simulink model "sm_forklift"  (R2021b)
settings: Solver=ode15s  StartTime=0.0  StopTime=53  MaxStep=1e-2  RelTol=1e-3  AbsTol=1e-3  EnableMultiTasking=on
model workspace: external: MATLAB File sm_forklift_parameters.m (data not in the file)
values from neighbouring files (symbols this model uses):
  g = 9.8    [sm_forklift_parameters.m]
undefined symbols (not defined in the file or in its folder): backRest, box, bump, chassis, fork, infPlane, main_mast, pulley, smiData, tire, top_mast, wheel, X, Y, Z
libraries: sm_lib x1413, nesl_utility x83, fl_lib x23, sm_backhoe_lib x6, SignalEditorBlockLib x1
(part 3 of 24)

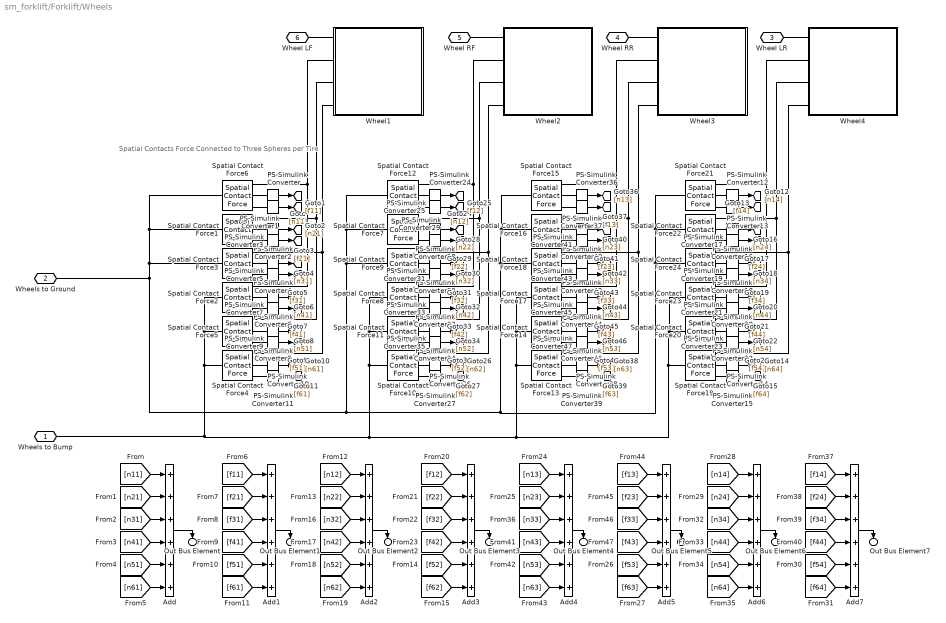
== system sm_forklift/Forklift/Wheels ==
  note: Spatial Contacts Force
      | Connected to Three Spheres per Tire
  Add{,1..7} (8 alike) : Sum  Inputs=++++++
  PS-Simulink Converter{,1..47} (48 alike) : nesl_utility/PS-Simulink Converter  PhysicalDomain=network_engine_domain  SubClassName=ps_output  LeftPortType=input  RightPortType=output  PseudoPeriodic=off  Frequencies=[]  Unit=inherit  AffineConversion=off
      settings: SourceProductBaseCode=PW,SS
  Spatial Contact Force{1..24} (24 alike) : sm_lib/Forces and Torques/Spatial Contact Force  CoefficientOfDynamicFriction=wDynamic  CoefficientOfStaticFriction=wStatic  SenseContactBaseRotation=off  SenseContactBaseTranslation=off  NormalDamping=wDamping  NormalDampingUnits=N/(m/s)  SenseContactFollowerRotation=off  SenseContactFollowerTranslation=off  SenseContactSignal=off  NormalStiffness=wStiffness  NormalStiffnessUnits=N/m  FrictionalCriticalVelocity=wCritical  FrictionalCriticalVelocityUnits=m/s  ZeroCrossDetectContactStartAndEnd=off  FrictionType=SmoothStickSlip  SenseFrictionalForceMagnitude=on  SenseNormalForceMagnitude=on  NormalForceType=SmoothSpringDamper  SenseNormalVelocity=off  SenseSeparationDistance=off  SenseTangentialVelocity=off  SenseTangentialVelocityMagnitude=off  NormalTransitionRegionWidth=wTransWidth  NormalTransitionRegionWidthUnits=mm
  Wheel1 : Subsystem  mask(Wheel){Rwheel=wRadius, Rtire=TireRadius, Raxle=wAxle, W=wWidth, Nc=wResolution, tireColor=TireColor, rhoTire=TireDensity, wheelColor=wColor, rhoWheel=wDensity}
      mask prompts: Rwheel "Wheel Radius (m)"; Rtire "Tire Radius (m)"; Raxle "Axle Radius (m)"; W "Wheel Width (m)"; Nc "Circle Resolution (pts/rev)"; tireColor "Tire Color"; rhoTire "Tire Density (kg/m^3)"; wheelColor "Wheel Color"; rhoWheel "Wheel Density (kg/m^3)"
      mask help:
      | Consists of the backhoe wheel assembly.
      |
      | Attachment points are:
      | A: The center of the wheel's axle.
      mask init:
      | % Circles
      | angles = (0:Nc)' * 2 * pi / Nc;
      | unit_circle = [cos(angles) sin(angles)];
      | unit_circle_cw = flipud(unit_circle);
      | 
      | % Wheel
      | wheelPoints = [Rwheel * unit_circle; Raxle * unit_circle_cw];
      | 
      | % Tire
      | tirePoints = [Rtire * unit_circle; Rwheel * unit_circle_cw];
      | 
      | % Rim
      | H = W*0.15;
      | k = H/(Rwheel^2);
      | vec = linspace(Rwheel,Raxle,10)';
      | rimPoints = [Raxle 0; vec  H-k*vec.^2];
      mask DialogControl ParameterTabVar0 Prompt: General
      mask DialogControl ParameterTabVar01 Prompt: Material Properties
      mask Display:
      | image(repmat(imread(fullfile(matlabroot,'toolbox','physmod','sm','smdemos','backhoe','images','sm_backhoe_wheel.png')),[1 1 3]));
      | port_label('lconn',1,'A');
  Wheel2 : Subsystem  mask(Wheel){Rwheel=wRadius, Rtire=TireRadius, Raxle=wAxle, W=wWidth, Nc=wResolution, tireColor=TireColor, rhoTire=TireDensity, wheelColor=wColor, rhoWheel=wDensity}
      mask prompts: Rwheel "Wheel Radius (m)"; Rtire "Tire Radius (m)"; Raxle "Axle Radius (m)"; W "Wheel Width (m)"; Nc "Circle Resolution (pts/rev)"; tireColor "Tire Color"; rhoTire "Tire Density (kg/m^3)"; wheelColor "Wheel Color"; rhoWheel "Wheel Density (kg/m^3)"
      mask help:
      | Consists of the backhoe wheel assembly.
      |
      | Attachment points are:
      | A: The center of the wheel's axle.
      mask init: same as sm_forklift/Forklift/Wheels/Wheel1
      mask DialogControl ParameterTabVar0 Prompt: General
      mask DialogControl ParameterTabVar01 Prompt: Material Properties
      mask Display:
      | image(repmat(imread(fullfile(matlabroot,'toolbox','physmod','sm','smdemos','backhoe','images','sm_backhoe_wheel.png')),[1 1 3]));
      | port_label('lconn',1,'A');
  Wheel3 : Subsystem  mask(Wheel){Rwheel=wRadius, Rtire=TireRadius, Raxle=wAxle, W=wWidth, Nc=wResolution, tireColor=TireColor, rhoTire=TireDensity, wheelColor=wColor, rhoWheel=wDensity}
      mask prompts: Rwheel "Wheel Radius (m)"; Rtire "Tire Radius (m)"; Raxle "Axle Radius (m)"; W "Wheel Width (m)"; Nc "Circle Resolution (pts/rev)"; tireColor "Tire Color"; rhoTire "Tire Density (kg/m^3)"; wheelColor "Wheel Color"; rhoWheel "Wheel Density (kg/m^3)"
      mask help:
      | Consists of the backhoe wheel assembly.
      |
      | Attachment points are:
      | A: The center of the wheel's axle.
      mask init: same as sm_forklift/Forklift/Wheels/Wheel1
      mask DialogControl ParameterTabVar0 Prompt: General
      mask DialogControl ParameterTabVar01 Prompt: Material Properties
      mask Display:
      | image(repmat(imread(fullfile(matlabroot,'toolbox','physmod','sm','smdemos','backhoe','images','sm_backhoe_wheel.png')),[1 1 3]));
      | port_label('lconn',1,'A');
  Wheel4 : Subsystem  mask(Wheel){Rwheel=wRadius, Rtire=TireRadius, Raxle=wAxle, W=wWidth, Nc=wResolution, tireColor=TireColor, rhoTire=TireDensity, wheelColor=wColor, rhoWheel=wDensity}
      mask prompts: Rwheel "Wheel Radius (m)"; Rtire "Tire Radius (m)"; Raxle "Axle Radius (m)"; W "Wheel Width (m)"; Nc "Circle Resolution (pts/rev)"; tireColor "Tire Color"; rhoTire "Tire Density (kg/m^3)"; wheelColor "Wheel Color"; rhoWheel "Wheel Density (kg/m^3)"
      mask help:
      | Consists of the backhoe wheel assembly.
      |
      | Attachment points are:
      | A: The center of the wheel's axle.
      mask init: same as sm_forklift/Forklift/Wheels/Wheel1
      mask DialogControl ParameterTabVar0 Prompt: General
      mask DialogControl ParameterTabVar01 Prompt: Material Properties
      mask Display:
      | image(repmat(imread(fullfile(matlabroot,'toolbox','physmod','sm','smdemos','backhoe','images','sm_backhoe_wheel.png')),[1 1 3]));
      | port_label('lconn',1,'A');
  Wheels to Bump : PMIOPort  Side=Right
  Wheels to Ground : PMIOPort  Port=2  Side=Right
  Wheel LR : PMIOPort  Port=3  Side=Left
  Wheel RR : PMIOPort  Port=4  Side=Left
  Wheel RF : PMIOPort  Port=5  Side=Left
  Wheel LF : PMIOPort  Port=6  Side=Left
  Out Bus Element : Outport  PortName=S  Element=NomalForce_WheelLF
  Out Bus Element1 : Outport  PortName=S  Element=FrictionalForce_WheelLF
  Out Bus Element2 : Outport  PortName=S  Element=NomalForce_WheelRF
  Out Bus Element3 : Outport  PortName=S  Element=FrictionalForce_WheelRF
  Out Bus Element4 : Outport  PortName=S  Element=NomalForce_WheelRR
  Out Bus Element5 : Outport  PortName=S  Element=FrictionalForce_WheelRR
  Out Bus Element6 : Outport  PortName=S  Element=NomalForce_WheelLR
  Out Bus Element7 : Outport  PortName=S  Element=FrictionalForce_WheelLR
  wires:
  PS-Simulink Converter/1 -> [n11]
  PS-Simulink Converter1/1 -> [f11]
  PS-Simulink Converter3/1 -> [f21]
  PS-Simulink Converter2/1 -> [n21]
  PS-Simulink Converter4/1 -> [n31]
  PS-Simulink Converter5/1 -> [f31]
  PS-Simulink Converter7/1 -> [f41]
  PS-Simulink Converter6/1 -> [n41]
  PS-Simulink Converter8/1 -> [n51]
  PS-Simulink Converter9/1 -> [f51]
  PS-Simulink Converter11/1 -> [f61]
  PS-Simulink Converter10/1 -> [n61]
  PS-Simulink Converter14/1 -> [n64]
  PS-Simulink Converter15/1 -> [f64]
  PS-Simulink Converter23/1 -> [f54]
  PS-Simulink Converter22/1 -> [n54]
  PS-Simulink Converter20/1 -> [n44]
  PS-Simulink Converter21/1 -> [f44]
  PS-Simulink Converter19/1 -> [f34]
  PS-Simulink Converter18/1 -> [n34]
  PS-Simulink Converter16/1 -> [n24]
  PS-Simulink Converter17/1 -> [f24]
  PS-Simulink Converter13/1 -> [f14]
  PS-Simulink Converter12/1 -> [n14]
  PS-Simulink Converter24/1 -> [n12]
  PS-Simulink Converter25/1 -> [f12]
  PS-Simulink Converter29/1 -> [f22]
  PS-Simulink Converter28/1 -> [n22]
  PS-Simulink Converter30/1 -> [n32]
  PS-Simulink Converter31/1 -> [f32]
  PS-Simulink Converter33/1 -> [f42]
  PS-Simulink Converter32/1 -> [n42]
  PS-Simulink Converter34/1 -> [n52]
  PS-Simulink Converter35/1 -> [f52]
  PS-Simulink Converter27/1 -> [f62]
  PS-Simulink Converter26/1 -> [n62]
  PS-Simulink Converter36/1 -> [n13]
  PS-Simulink Converter37/1 -> [f13]
  PS-Simulink Converter41/1 -> [f23]
  PS-Simulink Converter40/1 -> [n23]
  PS-Simulink Converter42/1 -> [n33]
  PS-Simulink Converter43/1 -> [f33]
  PS-Simulink Converter45/1 -> [f43]
  PS-Simulink Converter44/1 -> [n43]
  PS-Simulink Converter46/1 -> [n53]
  PS-Simulink Converter47/1 -> [f53]
  PS-Simulink Converter39/1 -> [f63]
  PS-Simulink Converter38/1 -> [n63]
  [n11] -> Add/1
  [n21] -> Add/2
  [n31] -> Add/3
  [n41] -> Add/4
  [n51] -> Add/5
  [n61] -> Add/6
  [f11] -> Add1/1
  [f31] -> Add1/3
  [f51] -> Add1/5
  [f21] -> Add1/2
  [f41] -> Add1/4
  [f61] -> Add1/6
  [n12] -> Add2/1
  [n22] -> Add2/2
  [n32] -> Add2/3
  [n42] -> Add2/4
  [n52] -> Add2/5
  [n62] -> Add2/6
  [f12] -> Add3/1
  [f22] -> Add3/2
  [f32] -> Add3/3
  [f42] -> Add3/4
  [f52] -> Add3/5
  [f62] -> Add3/6
  [f64] -> Add7/6
  [f54] -> Add7/5
  [f44] -> Add7/4
  [f34] -> Add7/3
  [f24] -> Add7/2
  [f14] -> Add7/1
  [n64] -> Add6/6
  [n54] -> Add6/5
  [n44] -> Add6/4
  [n34] -> Add6/3
  [n24] -> Add6/2
  [n14] -> Add6/1
  [f63] -> Add5/6
  [f43] -> Add5/4
  [f23] -> Add5/2
  [f53] -> Add5/5
  [f33] -> Add5/3
  [f13] -> Add5/1
  [n63] -> Add4/6
  [n53] -> Add4/5
  [n43] -> Add4/4
  [n33] -> Add4/3
  [n23] -> Add4/2
  [n13] -> Add4/1
  Add/1 -> Out Bus Element/1
  Add1/1 -> Out Bus Element1/1
  Add2/1 -> Out Bus Element2/1
  Add3/1 -> Out Bus Element3/1
  Add4/1 -> Out Bus Element4/1
  Add5/1 -> Out Bus Element5/1
  Add6/1 -> Out Bus Element6/1
  Add7/1 -> Out Bus Element7/1
  connections:
  Spatial Contact Force20/LConn1 -- Spatial Contact Force23/LConn1 -- Spatial Contact Force19/LConn1 -- Spatial Contact Force13/LConn1 -- Spatial Contact Force14/LConn1 -- Spatial Contact Force17/LConn1 -- Spatial Contact Force10/LConn1 -- Spatial Contact Force11/LConn1 -- Spatial Contact Force8/LConn1 -- Spatial Contact Force4/LConn1 -- Spatial Contact Force5/LConn1 -- Spatial Contact Force2/LConn1 -- Wheels to Bump/RConn1
  Spatial Contact Force22/LConn1 -- Spatial Contact Force21/LConn1 -- Spatial Contact Force24/LConn1 -- Spatial Contact Force18/LConn1 -- Spatial Contact Force16/LConn1 -- Spatial Contact Force15/LConn1 -- Spatial Contact Force9/LConn1 -- Spatial Contact Force12/LConn1 -- Spatial Contact Force7/LConn1 -- Spatial Contact Force3/LConn1 -- Spatial Contact Force1/LConn1 -- Spatial Contact Force6/LConn1 -- Wheels to Ground/RConn1
  Wheel4/LConn3 -- Spatial Contact Force22/RConn1 -- Spatial Contact Force20/RConn1
  Wheel1/LConn3 -- Spatial Contact Force5/RConn1 -- Spatial Contact Force1/RConn1
  Wheel3/LConn2 -- Spatial Contact Force17/RConn1 -- Spatial Contact Force15/RConn1
  Wheel4/LConn2 -- Spatial Contact Force23/RConn1 -- Spatial Contact Force21/RConn1
  Wheel1/LConn2 -- Spatial Contact Force2/RConn1 -- Spatial Contact Force6/RConn1
  Wheel4/LConn1 -- Wheel LR/RConn1
  Wheel2/LConn3 -- Spatial Contact Force11/RConn1 -- Spatial Contact Force7/RConn1
  Wheel4/LConn4 -- Spatial Contact Force24/RConn1 -- Spatial Contact Force19/RConn1
  Wheel1/LConn4 -- Spatial Contact Force4/RConn1 -- Spatial Contact Force3/RConn1
  Wheel2/LConn4 -- Spatial Contact Force10/RConn1 -- Spatial Contact Force9/RConn1
  Wheel3/LConn4 -- Spatial Contact Force18/RConn1 -- Spatial Contact Force13/RConn1
  Wheel2/LConn2 -- Spatial Contact Force12/RConn1 -- Spatial Contact Force8/RConn1
  Wheel3/LConn3 -- Spatial Contact Force16/RConn1 -- Spatial Contact Force14/RConn1
  Wheel2/LConn1 -- Wheel RF/RConn1
  Wheel1/LConn1 -- Wheel LF/RConn1
  Wheel3/LConn1 -- Wheel RR/RConn1
  Spatial Contact Force12/RConn2 -- PS-Simulink Converter24/LConn1
  Spatial Contact Force7/RConn2 -- PS-Simulink Converter28/LConn1
  Spatial Contact Force7/RConn3 -- PS-Simulink Converter29/LConn1
  Spatial Contact Force9/RConn2 -- PS-Simulink Converter30/LConn1
  Spatial Contact Force9/RConn3 -- PS-Simulink Converter31/LConn1
  Spatial Contact Force8/RConn2 -- PS-Simulink Converter32/LConn1
  Spatial Contact Force8/RConn3 -- PS-Simulink Converter33/LConn1
  Spatial Contact Force11/RConn2 -- PS-Simulink Converter34/LConn1
  Spatial Contact Force11/RConn3 -- PS-Simulink Converter35/LConn1
  PS-Simulink Converter/LConn1 -- Spatial Contact Force6/RConn2
  Spatial Contact Force6/RConn3 -- PS-Simulink Converter1/LConn1
  Spatial Contact Force1/RConn2 -- PS-Simulink Converter2/LConn1
  Spatial Contact Force3/RConn2 -- PS-Simulink Converter4/LConn1
  Spatial Contact Force3/RConn3 -- PS-Simulink Converter5/LConn1
  Spatial Contact Force1/RConn3 -- PS-Simulink Converter3/LConn1
  Spatial Contact Force2/RConn2 -- PS-Simulink Converter6/LConn1
  Spatial Contact Force2/RConn3 -- PS-Simulink Converter7/LConn1
  Spatial Contact Force5/RConn2 -- PS-Simulink Converter8/LConn1
  Spatial Contact Force5/RConn3 -- PS-Simulink Converter9/LConn1
  Spatial Contact Force4/RConn2 -- PS-Simulink Converter10/LConn1
  Spatial Contact Force4/RConn3 -- PS-Simulink Converter11/LConn1
  Spatial Contact Force19/RConn3 -- PS-Simulink Converter15/LConn1
  Spatial Contact Force19/RConn2 -- PS-Simulink Converter14/LConn1
  Spatial Contact Force20/RConn3 -- PS-Simulink Converter23/LConn1
  Spatial Contact Force23/RConn3 -- PS-Simulink Converter21/LConn1
  Spatial Contact Force23/RConn2 -- PS-Simulink Converter20/LConn1
  Spatial Contact Force24/RConn3 -- PS-Simulink Converter19/LConn1
  Spatial Contact Force22/RConn2 -- PS-Simulink Converter16/LConn1
  Spatial Contact Force22/RConn3 -- PS-Simulink Converter17/LConn1
  Spatial Contact Force21/RConn2 -- PS-Simulink Converter12/LConn1
  Spatial Contact Force21/RConn3 -- PS-Simulink Converter13/LConn1
  Spatial Contact Force20/RConn2 -- PS-Simulink Converter22/LConn1
  Spatial Contact Force24/RConn2 -- PS-Simulink Converter18/LConn1
  Spatial Contact Force12/RConn3 -- PS-Simulink Converter25/LConn1
  Spatial Contact Force10/RConn2 -- PS-Simulink Converter26/LConn1
  Spatial Contact Force10/RConn3 -- PS-Simulink Converter27/LConn1
  Spatial Contact Force18/RConn2 -- PS-Simulink Converter42/LConn1
  Spatial Contact Force14/RConn2 -- PS-Simulink Converter46/LConn1
  Spatial Contact Force15/RConn3 -- PS-Simulink Converter37/LConn1
  Spatial Contact Force15/RConn2 -- PS-Simulink Converter36/LConn1
  Spatial Contact Force16/RConn2 -- PS-Simulink Converter40/LConn1
  Spatial Contact Force17/RConn2 -- PS-Simulink Converter44/LConn1
  Spatial Contact Force16/RConn3 -- PS-Simulink Converter41/LConn1
  Spatial Contact Force17/RConn3 -- PS-Simulink Converter45/LConn1
  Spatial Contact Force14/RConn3 -- PS-Simulink Converter47/LConn1
  Spatial Contact Force13/RConn2 -- PS-Simulink Converter38/LConn1
  Spatial Contact Force13/RConn3 -- PS-Simulink Converter39/LConn1
  Spatial Contact Force18/RConn3 -- PS-Simulink Converter43/LConn1

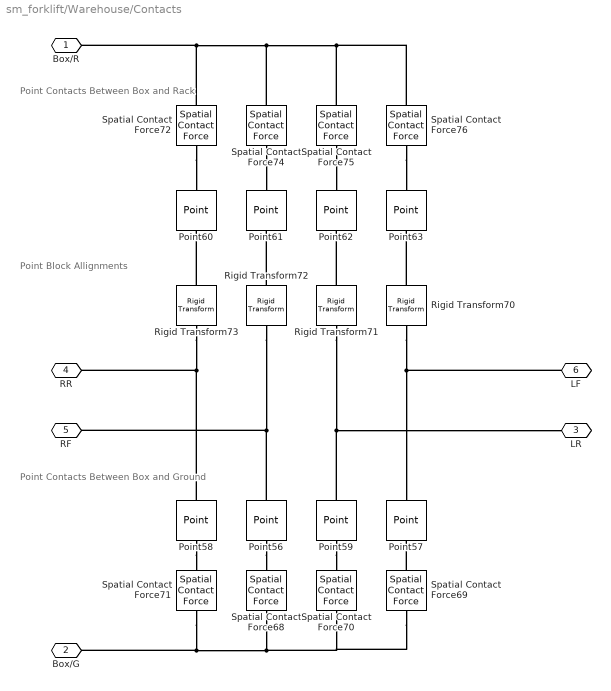
== system sm_forklift/Warehouse/Contacts ==
  note: Point Block Allignments
  note: Point Contacts
      | Between Box and
      | Ground
  note: Point Contacts
      | Between Box and
      | Rack
  Point{56..63} (8 alike) : sm_lib/Curves and Surfaces/Point  GraphicType=None  MarkerShape=Sphere  MarkerSize=10  GraphicVisPropType=SimpleVisualProperties  GraphicDiffuseColor=[0.5 0.5 0.5]  GraphicOpacity=1.0  GraphicSpecularColor=[0.5 0.5 0.5 1.0]  GraphicAmbientColor=[0.15 0.15 0.15 1.0]  GraphicEmissiveColor=[0.0 0.0 0.0 1.0]  GraphicShininess=75
      settings: SourceProductBaseCode=MS
  Rigid Transform70 : sm_lib/Frames and Transforms/Rigid Transform  TranslationMethod=StandardAxis  TranslationStandardOffset=0.2  TranslationLengthUnit=m  TranslationStandardAxis=+X  TranslationCartesianOffset=[0 0 0]  TranslationROffset=0  TranslationROffsetUnits=m  TranslationZOffset=0  TranslationZOffsetUnits=m  TranslationThetaOffset=0  TranslationThetaOffsetUnits=deg  RotationMethod=None  RotationAngleUnits=deg  RotationStandardAxis=+Z  RotationAngle=0.0  RotationArbitraryAxis=[0 0 1]  FollAlignAxisA=+X  BaseAlignAxisA=+Y  FollAlignAxisB=+Y  BaseAlignAxisB=+Z  RotationSequenceAxes=FollowerAxes  RotationSequence=XYX  RotationSequenceAngles=[0 0 0]  RotationSequenceAnglesUnits=deg  RotationMatrix=[1 0 0; 0 1 0; 0 0 1]
  Rigid Transform71 : sm_lib/Frames and Transforms/Rigid Transform  TranslationMethod=StandardAxis  TranslationStandardOffset=0.2  TranslationLengthUnit=m  TranslationStandardAxis=-X  TranslationCartesianOffset=[0 0 0]  TranslationROffset=0  TranslationROffsetUnits=m  TranslationZOffset=0  TranslationZOffsetUnits=m  TranslationThetaOffset=0  TranslationThetaOffsetUnits=deg  RotationMethod=None  RotationAngleUnits=deg  RotationStandardAxis=+Z  RotationAngle=0.0  RotationArbitraryAxis=[0 0 1]  FollAlignAxisA=+X  BaseAlignAxisA=+Y  FollAlignAxisB=+Y  BaseAlignAxisB=+Z  RotationSequenceAxes=FollowerAxes  RotationSequence=XYX  RotationSequenceAngles=[0 0 0]  RotationSequenceAnglesUnits=deg  RotationMatrix=[1 0 0; 0 1 0; 0 0 1]
  Rigid Transform72 : sm_lib/Frames and Transforms/Rigid Transform  TranslationMethod=StandardAxis  TranslationStandardOffset=0.2  TranslationLengthUnit=m  TranslationStandardAxis=+X  TranslationCartesianOffset=[0 0 0]  TranslationROffset=0  TranslationROffsetUnits=m  TranslationZOffset=0  TranslationZOffsetUnits=m  TranslationThetaOffset=0  TranslationThetaOffsetUnits=deg  RotationMethod=None  RotationAngleUnits=deg  RotationStandardAxis=+Z  RotationAngle=0.0  RotationArbitraryAxis=[0 0 1]  FollAlignAxisA=+X  BaseAlignAxisA=+Y  FollAlignAxisB=+Y  BaseAlignAxisB=+Z  RotationSequenceAxes=FollowerAxes  RotationSequence=XYX  RotationSequenceAngles=[0 0 0]  RotationSequenceAnglesUnits=deg  RotationMatrix=[1 0 0; 0 1 0; 0 0 1]
  Rigid Transform73 : sm_lib/Frames and Transforms/Rigid Transform  TranslationMethod=StandardAxis  TranslationStandardOffset=0.2  TranslationLengthUnit=m  TranslationStandardAxis=-X  TranslationCartesianOffset=[0 0 0]  TranslationROffset=0  TranslationROffsetUnits=m  TranslationZOffset=0  TranslationZOffsetUnits=m  TranslationThetaOffset=0  TranslationThetaOffsetUnits=deg  RotationMethod=None  RotationAngleUnits=deg  RotationStandardAxis=+Z  RotationAngle=0.0  RotationArbitraryAxis=[0 0 1]  FollAlignAxisA=+X  BaseAlignAxisA=+Y  FollAlignAxisB=+Y  BaseAlignAxisB=+Z  RotationSequenceAxes=FollowerAxes  RotationSequence=XYX  RotationSequenceAngles=[0 0 0]  RotationSequenceAnglesUnits=deg  RotationMatrix=[1 0 0; 0 1 0; 0 0 1]
  Spatial Contact Force{68..72,74..76} (8 alike) : sm_lib/Forces and Torques/Spatial Contact Force  CoefficientOfDynamicFriction=0.3  CoefficientOfStaticFriction=0.5  SenseContactBaseRotation=off  SenseContactBaseTranslation=off  NormalDamping=1e5  NormalDampingUnits=N/(m/s)  SenseContactFollowerRotation=off  SenseContactFollowerTranslation=off  SenseContactSignal=off  NormalStiffness=1e6  NormalStiffnessUnits=N/m  FrictionalCriticalVelocity=1e-3  FrictionalCriticalVelocityUnits=m/s  ZeroCrossDetectContactStartAndEnd=off  FrictionType=SmoothStickSlip  SenseFrictionalForceMagnitude=off  SenseNormalForceMagnitude=off  NormalForceType=SmoothSpringDamper  SenseNormalVelocity=off  SenseSeparationDistance=off  SenseTangentialVelocity=off  SenseTangentialVelocityMagnitude=off  NormalTransitionRegionWidth=1e-4  NormalTransitionRegionWidthUnits=m
  Box/R : PMIOPort  Side=Left
  Box/G : PMIOPort  Port=2  Side=Left
  LR : PMIOPort  Port=3  Side=Right
  RR : PMIOPort  Port=4  Side=Right
  RF : PMIOPort  Port=5  Side=Right
  LF : PMIOPort  Port=6  Side=Right
  connections:
  Spatial Contact Force71/LConn1 -- Box/G/RConn1 -- Spatial Contact Force69/LConn1 -- Spatial Contact Force70/LConn1 -- Spatial Contact Force68/LConn1
  Point56/LConn1 -- Rigid Transform72/LConn1 -- RF/RConn1
  Point58/RConn1 -- Spatial Contact Force71/RConn1
  Spatial Contact Force72/LConn1 -- Spatial Contact Force76/LConn1 -- Spatial Contact Force75/LConn1 -- Spatial Contact Force74/LConn1 -- Box/R/RConn1
  Point59/LConn1 -- Rigid Transform71/LConn1 -- LR/RConn1
  Spatial Contact Force72/RConn1 -- Point60/RConn1
  Rigid Transform71/RConn1 -- Point62/LConn1
  Point59/RConn1 -- Spatial Contact Force70/RConn1
  Rigid Transform70/RConn1 -- Point63/LConn1
  Rigid Transform73/RConn1 -- Point60/LConn1
  Spatial Contact Force69/RConn1 -- Point57/RConn1
  Point56/RConn1 -- Spatial Contact Force68/RConn1
  Spatial Contact Force75/RConn1 -- Point62/RConn1
  Spatial Contact Force76/RConn1 -- Point63/RConn1
  Rigid Transform70/LConn1 -- LF/RConn1 -- Point57/LConn1
  Point58/LConn1 -- Rigid Transform73/LConn1 -- RR/RConn1
  Rigid Transform72/RConn1 -- Point61/LConn1
  Spatial Contact Force74/RConn1 -- Point61/RConn1

== system sm_forklift/Warehouse/Lift Box ==
  Box : sm_lib/Body Elements/Brick Solid  GraphicAmbientColor=[0.15 0.15 0.15 1.0]  BasedOnType=Mass  BrickDimensions=boxDimensions  BrickDimensionUnits=m  CenterOfMass=[0 0 0]  CenterOfMassUnits=m  GraphicDiffuseColor=boxColor  Density=100  DensityUnits=kg/m^3  DoExposeReferenceFrame=off  GraphicEmissiveColor=[0.0 0.0 0.0 1.0]  ExportEntireGeometry=off  SerializedFrames=<Frames><Frame><Id>Frame1</Id><Value><Name>F1</Name><Origin><Source>GeometricFeature</Source><FeatureName>-z surface</FeatureName></Origin><PrimaryAxis><DefinedDirection>-Z</DefinedDirection><Source>GeometricFeature</Source><SourceDirection>+Z</SourceDirection><FeatureName>-z surface</FeatureName></PrimaryAxis><SecondaryAxis><DefinedDirection>+X</DefinedDirection><Source>ReferenceFrame</Source><SourceDirection>+X</SourceDirection><FeatureName></FeatureName></SecondaryAxis></Value></Frame></Frames>  MarkerShape=Sphere  MarkerSize=10  GraphicType=FromGeometry  InertiaType=CalculateFromGeometry  Mass=boxMass  MassUnits=kg  MomentsOfInertia=[1 1 1]  MomentsOfInertiaUnits=kg*m^2  GraphicOpacity=1.0  ProductsOfInertia=[0 0 0]  ProductsOfInertiaUnits=kg*m^2  GraphicShininess=75  GraphicSpecularColor=[0.5 0.5 0.5 1.0]  GraphicVisPropType=SimpleVisualProperties
  Box Base : sm_lib/Body Elements/File Solid  ExtGeomFileName=Palette_800x1200.step  UnitType=FromFile  ExtGeomFileUnits=m  StepReaderType=HEX  ExportConvexHullGeometry=off  InertiaType=CalculateFromGeometry  Mass=1  MassUnits=kg  CenterOfMass=[0 0 0]  CenterOfMassUnits=m  MomentsOfInertia=[1 1 1]  MomentsOfInertiaUnits=kg*m^2  ProductsOfInertia=[0 0 0]  ProductsOfInertiaUnits=kg*m^2  BasedOnType=Density  Density=bpDensity  DensityUnits=kg/m^3  DoExposeReferenceFrame=on  SerializedFrames=<Frames><Frame><Id>Frame1</Id><Value><Name>LR</Name><Origin><Source>GeometricFeature</Source><FeatureName>point 357</FeatureName></Origin><PrimaryAxis><DefinedDirection>+Z</DefinedDirection><Source>ReferenceFrame</Source><SourceDirection>+Z</SourceDirection><FeatureName></FeatureName></PrimaryAxis><SecondaryAxis><DefinedDirection>+X</DefinedDirection><Source>ReferenceFrame</Source><SourceDirection>+X</SourceDirection><FeatureName></FeatureName></SecondaryAxis></Value></Frame><Frame><Id>Frame2</Id><Value><Name>RR</Name><Origin><Source>GeometricFeature</Source><FeatureName>point 165</FeatureName></Origin><PrimaryAxis><DefinedDirection>+Z</DefinedDirection><Source>ReferenceFrame</Source><SourceDirection>+Z</SourceDirection><FeatureName></FeatureName></PrimaryAxis><SecondaryAxis><DefinedDirection>+X</DefinedDirection><Source>ReferenceFrame</Source><SourceDirection>+X</SourceDirection><FeatureName></FeatureName></SecondaryAxis></Value></Frame><Frame><Id>Frame3</Id><Value><Name>LF</Name><Origin><Source>GeometricFeature</Source><FeatureName>point 358</FeatureName></Origin><PrimaryAxis><DefinedDirection>+Z</DefinedDirection><Source>ReferenceFrame</Source><SourceDirection>+Z</SourceDirection><FeatureName></FeatureName></PrimaryAxis><SecondaryAxis><DefinedDirection>+X</DefinedDirection><Source>ReferenceFrame</Source><SourceDirection>+X</SourceDirection><FeatureName></FeatureName></SecondaryAxis></Value></Frame><Frame><Id>Frame4</Id><Value><Name>RF</Name><Origin><Source>GeometricFeature</Source><FeatureName>point 168</FeatureName></Origin><PrimaryAxis><DefinedDirection>+Z</DefinedDirection><Source>ReferenceFrame</Source><SourceDirection>+Z</SourceDirection><FeatureName></FeatureName></PrimaryAxis><SecondaryAxis><DefinedDirection>+X</DefinedDirection><Source>ReferenceFrame</Source><SourceDirection>+X</SourceDirection><FeatureName></FeatureName></SecondaryAxis></Value></Frame></Frames>  GraphicType=FromGeometry  MarkerShape=Sphere  MarkerSize=10  GraphicVisPropType=SimpleVisualProperties  GraphicDiffuseColor=bpColor  GraphicSpecularColor=[0.5 0.5 0.5 1.0]  GraphicAmbientColor=[0.15 0.15 0.15 1.0]  GraphicEmissiveColor=[0.0 0.0 0.0 1.0]  GraphicShininess=75  GraphicOpacity=1.0
  Brick Solid for Contact : sm_lib/Body Elements/Brick Solid  GraphicAmbientColor=[0.15 0.15 0.15 1.0]  BasedOnType=Density  BrickDimensions=[1200 800 40]  BrickDimensionUnits=mm  CenterOfMass=[0 0 0]  CenterOfMassUnits=m  GraphicDiffuseColor=[0.5 0.5 0.5]  Density=1000  DensityUnits=kg/m^3  DoExposeReferenceFrame=on  GraphicEmissiveColor=[0.0 0.0 0.0 1.0]  ExportEntireGeometry=on  SerializedFrames=<Frames/>  MarkerShape=Sphere  MarkerSize=10  GraphicType=None  InertiaType=CalculateFromGeometry  Mass=1  MassUnits=kg  MomentsOfInertia=[1 1 1]  MomentsOfInertiaUnits=kg*m^2  GraphicOpacity=1.0  ProductsOfInertia=[0 0 0]  ProductsOfInertiaUnits=kg*m^2  GraphicShininess=75  GraphicSpecularColor=[0.5 0.5 0.5 1.0]  GraphicVisPropType=SimpleVisualProperties
  LR : PMIOPort  Side=Left
  RR : PMIOPort  Port=2  Side=Left
  RF : PMIOPort  Port=3  Side=Left
  LF : PMIOPort  Port=4  Side=Left
  Box to Fork : PMIOPort  Port=5  Side=Right
  Ref : PMIOPort  Port=6  Side=Right
  connections:
  Box/LConn1 -- Brick Solid for Contact/RConn1 -- Ref/RConn1 -- Box Base/RConn1
  RF/RConn1 -- Box Base/LConn3
  RR/RConn1 -- Box Base/LConn2
  LR/RConn1 -- Box Base/LConn1
  Brick Solid for Contact/LConn1 -- Box to Fork/RConn1
  Box Base/RConn2 -- LF/RConn1

== system sm_forklift/Warehouse/Racks ==
  Rack 1 : Subsystem
  Rack 2 : Subsystem
  Rigid Transform : sm_lib/Frames and Transforms/Rigid Transform  TranslationMethod=Cartesian  TranslationStandardOffset=9  TranslationLengthUnit=m  TranslationStandardAxis=+Y  TranslationCartesianOffset=[-3.15 8 0]  TranslationROffset=0  TranslationROffsetUnits=m  TranslationZOffset=0  TranslationZOffsetUnits=m  TranslationThetaOffset=0  TranslationThetaOffsetUnits=deg  RotationMethod=None  RotationAngleUnits=deg  RotationStandardAxis=+Z  RotationAngle=0.0  RotationArbitraryAxis=[0 0 1]  FollAlignAxisA=+X  BaseAlignAxisA=+Y  FollAlignAxisB=+Y  BaseAlignAxisB=+Z  RotationSequenceAxes=FollowerAxes  RotationSequence=XYX  RotationSequenceAngles=[0 0 0]  RotationSequenceAnglesUnits=deg  RotationMatrix=[1 0 0; 0 1 0; 0 0 1]
  Rigid Transform1 : sm_lib/Frames and Transforms/Rigid Transform  TranslationMethod=StandardAxis  TranslationStandardOffset=16  TranslationLengthUnit=m  TranslationStandardAxis=-X  TranslationCartesianOffset=[0 0 0]  TranslationROffset=0  TranslationROffsetUnits=m  TranslationZOffset=0  TranslationZOffsetUnits=m  TranslationThetaOffset=0  TranslationThetaOffsetUnits=deg  RotationMethod=StandardAxis  RotationAngleUnits=deg  RotationStandardAxis=+Z  RotationAngle=90  RotationArbitraryAxis=[0 0 1]  FollAlignAxisA=+X  BaseAlignAxisA=+Y  FollAlignAxisB=+Y  BaseAlignAxisB=+Z  RotationSequenceAxes=FollowerAxes  RotationSequence=XYX  RotationSequenceAngles=[0 0 0]  RotationSequenceAnglesUnits=deg  RotationMatrix=[1 0 0; 0 1 0; 0 0 1]
  Rigid Transform67 : sm_lib/Frames and Transforms/Rigid Transform  TranslationMethod=StandardAxis  TranslationStandardOffset=1  TranslationLengthUnit=m  TranslationStandardAxis=-Y  TranslationCartesianOffset=[0 0 0]  TranslationROffset=0  TranslationROffsetUnits=m  TranslationZOffset=0  TranslationZOffsetUnits=m  TranslationThetaOffset=0  TranslationThetaOffsetUnits=deg  RotationMethod=StandardAxis  RotationAngleUnits=deg  RotationStandardAxis=+X  RotationAngle=-90  RotationArbitraryAxis=[0 0 1]  FollAlignAxisA=+X  BaseAlignAxisA=+Y  FollAlignAxisB=+Y  BaseAlignAxisB=+Z  RotationSequenceAxes=FollowerAxes  RotationSequence=XYX  RotationSequenceAngles=[0 0 0]  RotationSequenceAnglesUnits=deg  RotationMatrix=[1 0 0; 0 1 0; 0 0 1]
  W : PMIOPort  Side=Left
  Rack C : PMIOPort  Port=2  Side=Left
  connections:
  Rigid Transform/LConn1 -- Rigid Transform1/LConn1 -- Rigid Transform67/RConn1
  Rigid Transform/RConn1 -- Rack 1/LConn1
  Rack 2/LConn1 -- Rigid Transform1/RConn1
  Rack C/RConn1 -- Rack 1/LConn2
  Rigid Transform67/LConn1 -- W/RConn1

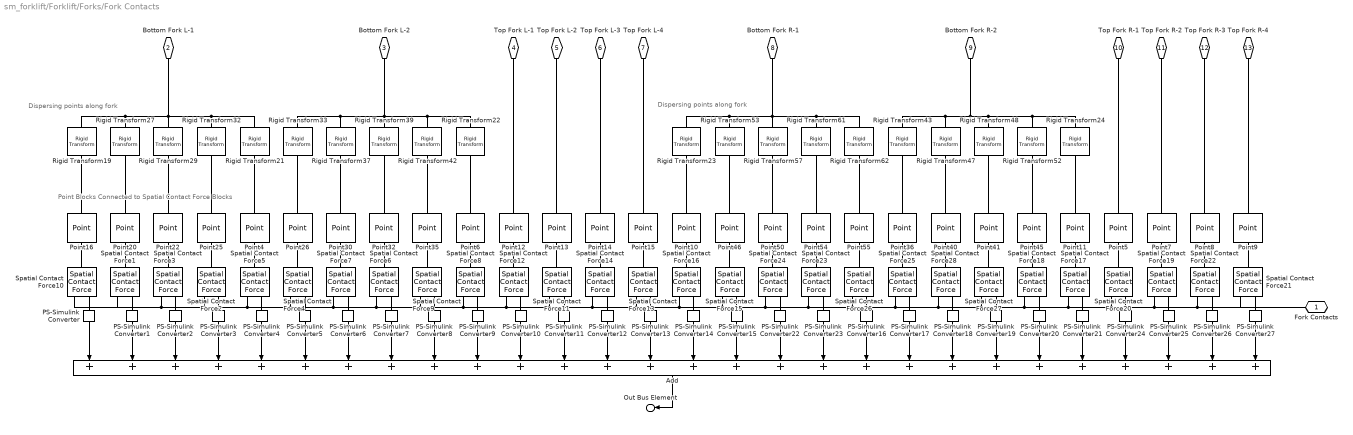
== system sm_forklift/Forklift/Forks/Fork Contacts ==
  note: Point Blocks Connected to Spatial Contact Force Blocks
  note: Dispersing points along fork
  note: Dispersing points along fork
  Add : Sum  Inputs=++++++++++++++++++++++++++++
  PS-Simulink Converter{,1..27} (28 alike) : nesl_utility/PS-Simulink Converter  PhysicalDomain=network_engine_domain  SubClassName=ps_output  LeftPortType=input  RightPortType=output  PseudoPeriodic=off  Frequencies=[]  Unit=inherit  AffineConversion=off
      settings: SourceProductBaseCode=PW,SS
  Point{4..16,20,22,25..26,30,32,35..36,40..41,45..46,50,54..55} (28 alike) : sm_lib/Curves and Surfaces/Point  GraphicType=None  MarkerShape=Sphere  MarkerSize=10  GraphicVisPropType=SimpleVisualProperties  GraphicDiffuseColor=[0 0.5 0]  GraphicOpacity=1.0  GraphicSpecularColor=[0.5 0.5 0.5 1.0]  GraphicAmbientColor=[0.15 0.15 0.15 1.0]  GraphicEmissiveColor=[0.0 0.0 0.0 1.0]  GraphicShininess=75
      settings: SourceProductBaseCode=MS
  Rigid Transform{19,33,43,53} (4 alike) : sm_lib/Frames and Transforms/Rigid Transform  TranslationMethod=StandardAxis  TranslationStandardOffset=200  TranslationLengthUnit=mm  TranslationStandardAxis=+X  TranslationCartesianOffset=[0 0 0]  TranslationROffset=0  TranslationROffsetUnits=m  TranslationZOffset=0  TranslationZOffsetUnits=m  TranslationThetaOffset=0  TranslationThetaOffsetUnits=deg  RotationMethod=None  RotationAngleUnits=deg  RotationStandardAxis=+Z  RotationAngle=0.0  RotationArbitraryAxis=[0 0 1]  FollAlignAxisA=+X  BaseAlignAxisA=+Y  FollAlignAxisB=+Y  BaseAlignAxisB=+Z  RotationSequenceAxes=FollowerAxes  RotationSequence=XYX  RotationSequenceAngles=[0 0 0]  RotationSequenceAnglesUnits=deg  RotationMatrix=[1 0 0; 0 1 0; 0 0 1]
  Rigid Transform{21..24} (4 alike) : sm_lib/Frames and Transforms/Rigid Transform  TranslationMethod=StandardAxis  TranslationStandardOffset=100  TranslationLengthUnit=mm  TranslationStandardAxis=+X  TranslationCartesianOffset=[0 0 0]  TranslationROffset=0  TranslationROffsetUnits=m  TranslationZOffset=0  TranslationZOffsetUnits=m  TranslationThetaOffset=0  TranslationThetaOffsetUnits=deg  RotationMethod=None  RotationAngleUnits=deg  RotationStandardAxis=+Z  RotationAngle=0.0  RotationArbitraryAxis=[0 0 1]  FollAlignAxisA=+X  BaseAlignAxisA=+Y  FollAlignAxisB=+Y  BaseAlignAxisB=+Z  RotationSequenceAxes=FollowerAxes  RotationSequence=XYX  RotationSequenceAngles=[0 0 0]  RotationSequenceAnglesUnits=deg  RotationMatrix=[1 0 0; 0 1 0; 0 0 1]
  Rigid Transform{27,37,47,57} (4 alike) : sm_lib/Frames and Transforms/Rigid Transform  TranslationMethod=StandardAxis  TranslationStandardOffset=600  TranslationLengthUnit=mm  TranslationStandardAxis=+X  TranslationCartesianOffset=[0 0 0]  TranslationROffset=0  TranslationROffsetUnits=m  TranslationZOffset=0  TranslationZOffsetUnits=m  TranslationThetaOffset=0  TranslationThetaOffsetUnits=deg  RotationMethod=None  RotationAngleUnits=deg  RotationStandardAxis=+Z  RotationAngle=0.0  RotationArbitraryAxis=[0 0 1]  FollAlignAxisA=+X  BaseAlignAxisA=+Y  FollAlignAxisB=+Y  BaseAlignAxisB=+Z  RotationSequenceAxes=FollowerAxes  RotationSequence=XYX  RotationSequenceAngles=[0 0 0]  RotationSequenceAnglesUnits=deg  RotationMatrix=[1 0 0; 0 1 0; 0 0 1]
  Rigid Transform{29,39,48,61} (4 alike) : sm_lib/Frames and Transforms/Rigid Transform  TranslationMethod=StandardAxis  TranslationStandardOffset=800  TranslationLengthUnit=mm  TranslationStandardAxis=+X  TranslationCartesianOffset=[0 0 0]  TranslationROffset=0  TranslationROffsetUnits=m  TranslationZOffset=0  TranslationZOffsetUnits=m  TranslationThetaOffset=0  TranslationThetaOffsetUnits=deg  RotationMethod=None  RotationAngleUnits=deg  RotationStandardAxis=+Z  RotationAngle=0.0  RotationArbitraryAxis=[0 0 1]  FollAlignAxisA=+X  BaseAlignAxisA=+Y  FollAlignAxisB=+Y  BaseAlignAxisB=+Z  RotationSequenceAxes=FollowerAxes  RotationSequence=XYX  RotationSequenceAngles=[0 0 0]  RotationSequenceAnglesUnits=deg  RotationMatrix=[1 0 0; 0 1 0; 0 0 1]
  Rigid Transform{32,42,52,62} (4 alike) : sm_lib/Frames and Transforms/Rigid Transform  TranslationMethod=StandardAxis  TranslationStandardOffset=1100  TranslationLengthUnit=mm  TranslationStandardAxis=+X  TranslationCartesianOffset=[0 0 0]  TranslationROffset=0  TranslationROffsetUnits=m  TranslationZOffset=0  TranslationZOffsetUnits=m  TranslationThetaOffset=0  TranslationThetaOffsetUnits=deg  RotationMethod=None  RotationAngleUnits=deg  RotationStandardAxis=+Z  RotationAngle=0.0  RotationArbitraryAxis=[0 0 1]  FollAlignAxisA=+X  BaseAlignAxisA=+Y  FollAlignAxisB=+Y  BaseAlignAxisB=+Z  RotationSequenceAxes=FollowerAxes  RotationSequence=XYX  RotationSequenceAngles=[0 0 0]  RotationSequenceAnglesUnits=deg  RotationMatrix=[1 0 0; 0 1 0; 0 0 1]
  Spatial Contact Force{1..28} (28 alike) : sm_lib/Forces and Torques/Spatial Contact Force  CoefficientOfDynamicFriction=fDynamic  CoefficientOfStaticFriction=fStatic  SenseContactBaseRotation=off  SenseContactBaseTranslation=off  NormalDamping=fDamping  NormalDampingUnits=N/(m/s)  SenseContactFollowerRotation=off  SenseContactFollowerTranslation=off  SenseContactSignal=off  NormalStiffness=fStiffness  NormalStiffnessUnits=N/m  FrictionalCriticalVelocity=fCritical  FrictionalCriticalVelocityUnits=m/s  ZeroCrossDetectContactStartAndEnd=off  FrictionType=SmoothStickSlip  SenseFrictionalForceMagnitude=off  SenseNormalForceMagnitude=on  NormalForceType=SmoothSpringDamper  SenseNormalVelocity=off  SenseSeparationDistance=off  SenseTangentialVelocity=off  SenseTangentialVelocityMagnitude=off  NormalTransitionRegionWidth=fTransWidth  NormalTransitionRegionWidthUnits=m
  Fork Contacts : PMIOPort  Side=Right
  Bottom Fork L-1 : PMIOPort  Port=2  Side=Left
  Bottom Fork L-2 : PMIOPort  Port=3  Side=Left
  Top Fork L-1 : PMIOPort  Port=4  Side=Left
  Top Fork L-2 : PMIOPort  Port=5  Side=Left
  Top Fork L-3 : PMIOPort  Port=6  Side=Left
  Top Fork L-4 : PMIOPort  Port=7  Side=Left
  Bottom Fork R-1 : PMIOPort  Port=8  Side=Left
  Bottom Fork R-2 : PMIOPort  Port=9  Side=Left
  Top Fork R-1 : PMIOPort  Port=10  Side=Left
  Top Fork R-2 : PMIOPort  Port=11  Side=Left
  Top Fork R-3 : PMIOPort  Port=12  Side=Left
  Top Fork R-4 : PMIOPort  Port=13  Side=Left
  Out Bus Element : Outport  PortName=S  Element=ContactForceBetweenForks&Box
  wires:
  PS-Simulink Converter27/1 -> Add/28
  PS-Simulink Converter26/1 -> Add/27
  PS-Simulink Converter25/1 -> Add/26
  PS-Simulink Converter24/1 -> Add/25
  PS-Simulink Converter21/1 -> Add/24
  PS-Simulink Converter20/1 -> Add/23
  PS-Simulink Converter19/1 -> Add/22
  PS-Simulink Converter18/1 -> Add/21
  PS-Simulink Converter17/1 -> Add/20
  PS-Simulink Converter16/1 -> Add/19
  PS-Simulink Converter23/1 -> Add/18
  PS-Simulink Converter22/1 -> Add/17
  PS-Simulink Converter15/1 -> Add/16
  PS-Simulink Converter14/1 -> Add/15
  PS-Simulink Converter13/1 -> Add/14
  PS-Simulink Converter12/1 -> Add/13
  PS-Simulink Converter11/1 -> Add/12
  PS-Simulink Converter10/1 -> Add/11
  PS-Simulink Converter9/1 -> Add/10
  PS-Simulink Converter8/1 -> Add/9
  PS-Simulink Converter7/1 -> Add/8
  PS-Simulink Converter6/1 -> Add/7
  PS-Simulink Converter5/1 -> Add/6
  PS-Simulink Converter4/1 -> Add/5
  PS-Simulink Converter3/1 -> Add/4
  PS-Simulink Converter2/1 -> Add/3
  PS-Simulink Converter1/1 -> Add/2
  PS-Simulink Converter/1 -> Add/1
  Add/1 -> Out Bus Element/1
  connections:
  Spatial Contact Force1/LConn1 -- Point20/RConn1
  Spatial Contact Force15/LConn1 -- Point46/RConn1
  Spatial Contact Force5/LConn1 -- Point4/RConn1
  Spatial Contact Force26/RConn1 -- Spatial Contact Force25/RConn1 -- Spatial Contact Force28/RConn1 -- Spatial Contact Force27/RConn1 -- Spatial Contact Force18/RConn1 -- Spatial Contact Force17/RConn1 -- Spatial Contact Force20/RConn1 -- Spatial Contact Force19/RConn1 -- Spatial Contact Force22/RConn1 -- Spatial Contact Force21/RConn1 -- Fork Contacts/RConn1 -- Spatial Contact Force23/RConn1 -- Spatial Contact Force24/RConn1 -- Spatial Contact Force15/RConn1 -- Spatial Contact Force16/RConn1 -- Spatial Contact Force13/RConn1 -- Spatial Contact Force14/RConn1 -- Spatial Contact Force11/RConn1 -- Spatial Contact Force12/RConn1 -- Spatial Contact Force8/RConn1 -- Spatial Contact Force9/RConn1 -- Spatial Contact Force6/RConn1 -- Spatial Contact Force7/RConn1 -- Spatial Contact Force4/RConn1 -- Spatial Contact Force5/RConn1 -- Spatial Contact Force2/RConn1 -- Spatial Contact Force3/RConn1 -- Spatial Contact Force1/RConn1 -- Spatial Contact Force10/RConn1
  Spatial Contact Force28/LConn1 -- Point40/RConn1
  Spatial Contact Force23/LConn1 -- Point54/RConn1
  Rigid Transform39/RConn1 -- Point32/LConn1
  Rigid Transform62/RConn1 -- Point55/LConn1
  Top Fork L-2/RConn1 -- Point13/LConn1
  Rigid Transform57/RConn1 -- Point50/LConn1
  Rigid Transform37/RConn1 -- Point30/LConn1
  Rigid Transform27/RConn1 -- Point20/LConn1
  Spatial Contact Force6/LConn1 -- Point32/RConn1
  Spatial Contact Force24/LConn1 -- Point50/RConn1
  Spatial Contact Force19/LConn1 -- Point7/RConn1
  Top Fork L-1/RConn1 -- Point12/LConn1
  Rigid Transform47/RConn1 -- Point40/LConn1
  Spatial Contact Force16/LConn1 -- Point10/RConn1
  Spatial Contact Force14/LConn1 -- Point14/RConn1
  Rigid Transform61/RConn1 -- Point54/LConn1
  Top Fork R-2/RConn1 -- Point7/LConn1
  Spatial Contact Force20/LConn1 -- Point5/RConn1
  Rigid Transform32/RConn1 -- Point25/LConn1
  Rigid Transform22/RConn1 -- Point6/LConn1
  Spatial Contact Force4/LConn1 -- Point26/RConn1
  Top Fork L-4/RConn1 -- Point15/LConn1
  Rigid Transform19/RConn1 -- Point16/LConn1
  Spatial Contact Force2/LConn1 -- Point25/RConn1
  Spatial Contact Force11/LConn1 -- Point13/RConn1
  Spatial Contact Force26/LConn1 -- Point55/RConn1
  Spatial Contact Force25/LConn1 -- Point36/RConn1
  Spatial Contact Force17/LConn1 -- Point11/RConn1
  Spatial Contact Force8/LConn1 -- Point6/RConn1
  Top Fork R-1/RConn1 -- Point5/LConn1
  Spatial Contact Force18/LConn1 -- Point45/RConn1
  Rigid Transform42/RConn1 -- Point35/LConn1
  Spatial Contact Force21/LConn1 -- Point9/RConn1
  Rigid Transform48/RConn1 -- Point41/LConn1
  Rigid Transform52/LConn1 -- Bottom Fork R-2/RConn1 -- Rigid Transform47/LConn1 -- Rigid Transform43/LConn1 -- Rigid Transform48/LConn1 -- Rigid Transform24/LConn1
  Rigid Transform53/RConn1 -- Point46/LConn1
  Rigid Transform33/RConn1 -- Point26/LConn1
  Spatial Contact Force12/LConn1 -- Point12/RConn1
  Top Fork R-4/RConn1 -- Point9/LConn1
  Rigid Transform43/RConn1 -- Point36/LConn1
  Rigid Transform29/RConn1 -- Point22/LConn1
  Point16/RConn1 -- Spatial Contact Force10/LConn1
  Spatial Contact Force7/LConn1 -- Point30/RConn1
  Spatial Contact Force22/LConn1 -- Point8/RConn1
  Spatial Contact Force3/LConn1 -- Point22/RConn1
  Spatial Contact Force13/LConn1 -- Point15/RConn1
  Rigid Transform52/RConn1 -- Point45/LConn1
  Spatial Contact Force27/LConn1 -- Point41/RConn1
  Spatial Contact Force9/LConn1 -- Point35/RConn1
  Rigid Transform23/RConn1 -- Point10/LConn1
  Top Fork L-3/RConn1 -- Point14/LConn1
  Top Fork R-3/RConn1 -- Point8/LConn1
  Rigid Transform19/LConn1 -- Rigid Transform27/LConn1 -- Rigid Transform21/LConn1 -- Rigid Transform32/LConn1 -- Bottom Fork L-1/RConn1 -- Rigid Transform29/LConn1
  Rigid Transform21/RConn1 -- Point4/LConn1
  Rigid Transform42/LConn1 -- Bottom Fork L-2/RConn1 -- Rigid Transform33/LConn1 -- Rigid Transform37/LConn1 -- Rigid Transform39/LConn1 -- Rigid Transform22/LConn1
  Rigid Transform53/LConn1 -- Rigid Transform62/LConn1 -- Rigid Transform61/LConn1 -- Bottom Fork R-1/RConn1 -- Rigid Transform57/LConn1 -- Rigid Transform23/LConn1
  Rigid Transform24/RConn1 -- Point11/LConn1
  PS-Simulink Converter/LConn1 -- Spatial Contact Force10/RConn2
  Spatial Contact Force1/RConn2 -- PS-Simulink Converter1/LConn1
  Spatial Contact Force2/RConn2 -- PS-Simulink Converter3/LConn1
  Spatial Contact Force3/RConn2 -- PS-Simulink Converter2/LConn1
  Spatial Contact Force6/RConn2 -- PS-Simulink Converter7/LConn1
  Spatial Contact Force7/RConn2 -- PS-Simulink Converter6/LConn1
  Spatial Contact Force5/RConn2 -- PS-Simulink Converter4/LConn1
  Spatial Contact Force4/RConn2 -- PS-Simulink Converter5/LConn1
  Spatial Contact Force21/RConn2 -- PS-Simulink Converter27/LConn1
  Spatial Contact Force22/RConn2 -- PS-Simulink Converter26/LConn1
  Spatial Contact Force19/RConn2 -- PS-Simulink Converter25/LConn1
  Spatial Contact Force20/RConn2 -- PS-Simulink Converter24/LConn1
  Spatial Contact Force17/RConn2 -- PS-Simulink Converter21/LConn1
  Spatial Contact Force18/RConn2 -- PS-Simulink Converter20/LConn1
  Spatial Contact Force27/RConn2 -- PS-Simulink Converter19/LConn1
  Spatial Contact Force28/RConn2 -- PS-Simulink Converter18/LConn1
  Spatial Contact Force25/RConn2 -- PS-Simulink Converter17/LConn1
  Spatial Contact Force26/RConn2 -- PS-Simulink Converter16/LConn1
  Spatial Contact Force23/RConn2 -- PS-Simulink Converter23/LConn1
  Spatial Contact Force24/RConn2 -- PS-Simulink Converter22/LConn1
  Spatial Contact Force15/RConn2 -- PS-Simulink Converter15/LConn1
  Spatial Contact Force16/RConn2 -- PS-Simulink Converter14/LConn1
  Spatial Contact Force13/RConn2 -- PS-Simulink Converter13/LConn1
  Spatial Contact Force14/RConn2 -- PS-Simulink Converter12/LConn1
  Spatial Contact Force11/RConn2 -- PS-Simulink Converter11/LConn1
  Spatial Contact Force12/RConn2 -- PS-Simulink Converter10/LConn1
  Spatial Contact Force8/RConn2 -- PS-Simulink Converter9/LConn1
  Spatial Contact Force9/RConn2 -- PS-Simulink Converter8/LConn1
